simulink model "matsim_func"  (R2022b)
settings: Solver=FixedStepAuto  StartTime=0.0  StopTime=10  FixedStep=0.01  MaxStep=0.1  RelTol=1e-3
settings Model: Creator=Brigosha_Guest  LastModifiedBy=Brigosha_Guest

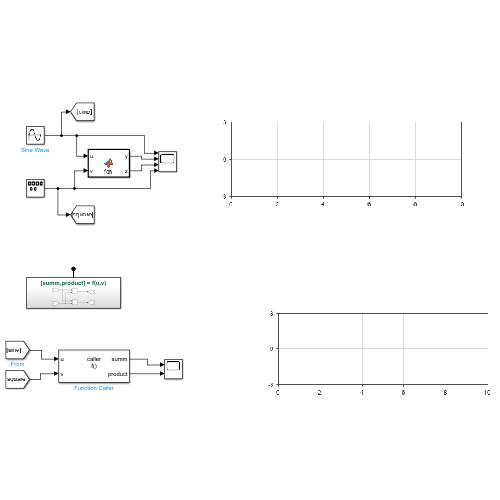
[thumbnail: Simulink's stored preview of the top-level diagram]
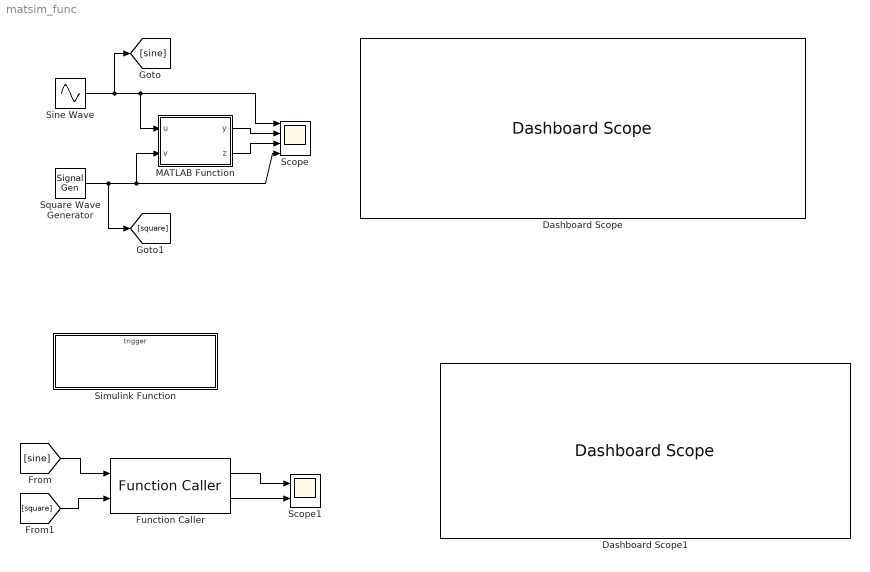
== system matsim_func ==
  Dashboard Scope : DashboardScope  ScaleAtStop=off  UpdateMode=Scroll
  Dashboard Scope1 : DashboardScope  ScaleAtStop=off  UpdateMode=Scroll
  Function Caller : FunctionCaller  FunctionPrototype=[summ,product] = f(u,v)  InputArgumentSpecifications=<Enter example>  OutputArgumentSpecifications=<Enter example>
  MATLAB Function : MATLAB Function  TreatAsAtomicUnit=on
  Scope : Scope  NumInputPorts=4
  Scope1 : Scope  NumInputPorts=2
  Simulink Function : Subsystem  TreatAsAtomicUnit=on
  Sine Wave : Sin  SampleTime=0
  Square Wave Generator : SignalGenerator  WaveForm=square
  wires:
  Sine Wave/1 -> [sine], MATLAB Function/1(u), Scope/1
  MATLAB Function/1(y) -> Scope/2
  Square Wave Generator/1 -> [square], Scope/4, MATLAB Function/2(v)
  MATLAB Function/2(z) -> Scope/3
  [sine] -> Function Caller/1
  [square] -> Function Caller/2
  Function Caller/1 -> Scope1/1
  Function Caller/2 -> Scope1/2

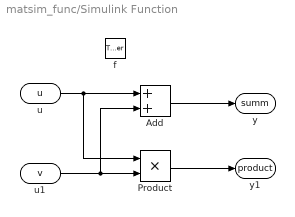
== system matsim_func/Simulink Function ==
  f : TriggerPort  TriggerType=function-call  IsSimulinkFunction=on  FunctionName=f  FunctionVisibility=scoped  VariantControl=(inherit)
  Add : Sum
  Product : Product
  u : ArgIn  DisableCoverage=on  ArgumentName=u
  u1 : ArgIn  DisableCoverage=on  Port=2  ArgumentName=v
  y : ArgOut  DisableCoverage=on  ArgumentName=summ
  y1 : ArgOut  DisableCoverage=on  Port=2  ArgumentName=product
  wires:
  u/1 -> Product/1, Add/1
  Add/1 -> y/1
  u1/1 -> Product/2, Add/2
  Product/1 -> y1/1

== matlab function matsim_func/MATLAB Function ==
  data: u input; y output; v input; z output
function [y,z] = fcn(u,v)
y=u*v;
z=u+v;
